simulink model "DC_motor_control_project"  (R2025a)
settings: Solver=VariableStepAuto  StartTime=0.0  StopTime=10.0  RelTol=1e-3
libraries: simulink x1, spsTriangleGeneratorLib x1
settings Model: Creator=HP  LastModifiedBy=HP

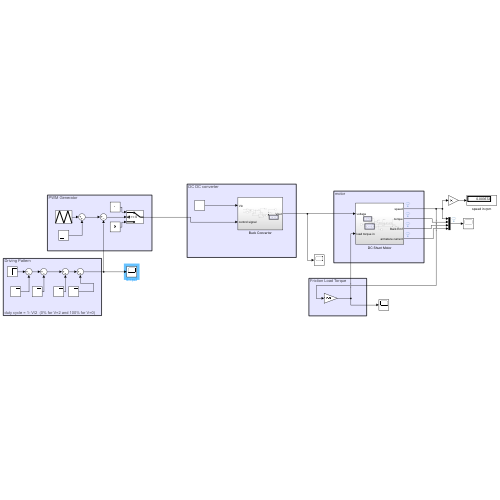
[thumbnail: Simulink's stored preview of the top-level diagram]
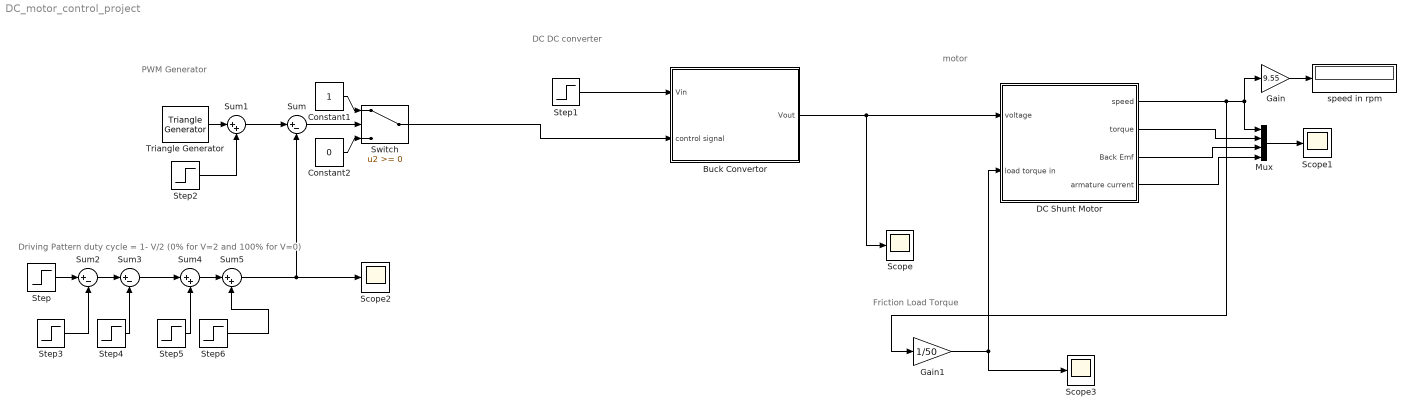
== system DC_motor_control_project ==
  note: motor
  note: Driving Pattern
      |
      |
      |
      |
      |
      |
      |
      |
      |
      |
      | duty cycle = 1- V/2  (0% for V=2 and 100% for V=0)
  note: PWM Generator
  note: DC DC converter
  note: Friction Load Torque
  Buck Convertor : Subsystem
  Constant1 : Constant
  Constant2 : Constant  Value=0
  DC Shunt Motor : Subsystem
  Gain : Gain  Gain=9.55
  Gain1 : Gain  Gain=1/50
  Mux : Mux
  Scope{,1..3} (4 alike) : Scope
      Scope settings: ActiveDisplayYMinimum=-42.370071739541189  ActiveDisplayYMaximum=281.05665253551075  DataLoggingVariableName=ScopeData4
      Scope1 settings: ActiveDisplayYMinimum=-124.79095  ActiveDisplayYMaximum=744.9713
      Scope2 settings: ActiveDisplayYMinimum=-0.24999999999999994  ActiveDisplayYMaximum=2.25  DataLoggingVariableName=ScopeData5
      Scope3 settings: ActiveDisplayYMinimum=-1.8285380504812083  ActiveDisplayYMaximum=16.456842454330879  DataLoggingVariableName=ScopeData6
  Step : Step  Time=0  SampleTime=0
  Step1 : Step  Time=0  After=240  SampleTime=0
  Step2 : Step  Time=0  SampleTime=0
  Step3 : Step  After=0.5  SampleTime=0
  Step4 : Step  Time=2  After=0.5  SampleTime=0
  Step5 : Step  Time=3  After=1.5  SampleTime=0
  Step6 : Step  Time=4  After=0.5  SampleTime=0
  Sum : Sum  Inputs=|+-
  Sum1 : Sum  Inputs=|++
  Sum2 : Sum  Inputs=|+-
  Sum3 : Sum  Inputs=|+-
  Sum4 : Sum  Inputs=|++
  Sum5 : Sum  Inputs=|++
  Switch : Switch  SaturateOnIntegerOverflow=off  InputSameDT=off
  Triangle Generator : spsTriangleGeneratorLib/Triangle Generator  Freq=1e3  Phase=0  Ts=0
  speed in rpm : Display
  wires:
  DC Shunt Motor/4(armature current) -> Mux/4
  DC Shunt Motor/1(speed) -> Gain1/1, Mux/1, Gain/1
  Step1/1 -> Buck Convertor/1(Vin)
  DC Shunt Motor/3(Back Emf) -> Mux/3
  Triangle Generator/1 -> Sum1/1
  Step3/1 -> Sum2/2
  Buck Convertor/1(Vout) -> Scope/1, DC Shunt Motor/1(voltage)
  Step6/1 -> Sum5/2
  Step/1 -> Sum2/1
  Gain/1 -> speed in rpm/1
  Sum3/1 -> Sum4/1
  Sum4/1 -> Sum5/1
  Mux/1 -> Scope1/1
  Constant1/1 -> Switch/1
  Step2/1 -> Sum1/2
  Sum2/1 -> Sum3/1
  Gain1/1 -> DC Shunt Motor/2(load torque in), Scope3/1
  Switch/1 -> Buck Convertor/2(control signal)
  Step5/1 -> Sum4/2
  Constant2/1 -> Switch/3
  Sum5/1 -> Scope2/1, Sum/2
  Sum/1 -> Switch/2
  Step4/1 -> Sum3/2
  Sum1/1 -> Sum/1
  DC Shunt Motor/2(torque) -> Mux/2

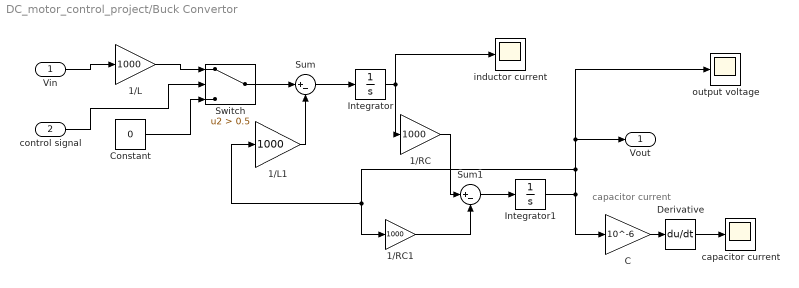
== system DC_motor_control_project/Buck Convertor ==
  note: capacitor current
  Vin : Inport
  control signal : Inport  Port=2
  1/L : Gain  Gain=1000
  1/L1 : Gain  Gain=1000
  1/RC : Gain  Gain=1000
  1/RC1 : Gain  Gain=1000
  C : Gain  Gain=10^-6
  Constant : Constant  Value=0
  Derivative : Derivative
  Integrator : Integrator
  Integrator1 : Integrator
  Sum : Sum  Inputs=|+-
  Sum1 : Sum  Inputs=|+-
  Switch : Switch  Criteria=u2 > Threshold  Threshold=0.5  SaturateOnIntegerOverflow=off  InputSameDT=off
  capacitor current : Scope
      settings: ActiveDisplayYMinimum=-0.14224  ActiveDisplayYMaximum=0.11943  DataLoggingVariableName=ScopeData2
  inductor current : Scope
      settings: ActiveDisplayYMinimum=-52.93589  ActiveDisplayYMaximum=290.861
  output voltage : Scope
      settings: ActiveDisplayYMinimum=-30  ActiveDisplayYMaximum=270  DataLoggingVariableName=ScopeData7
  Vout : Outport
  wires:
  1/L/1 -> Switch/1
  Switch/1 -> Sum/1
  Vin/1 -> 1/L/1
  1/L1/1 -> Sum/2
  Constant/1 -> Switch/3
  Sum/1 -> Integrator/1
  Integrator/1 -> inductor current/1, 1/RC/1
  1/RC/1 -> Sum1/1
  1/RC1/1 -> Sum1/2
  Sum1/1 -> Integrator1/1
  Integrator1/1 -> C/1, 1/L1/1, 1/RC1/1, output voltage/1, Vout/1
  control signal/1 -> Switch/2
  C/1 -> Derivative/1
  Derivative/1 -> capacitor current/1

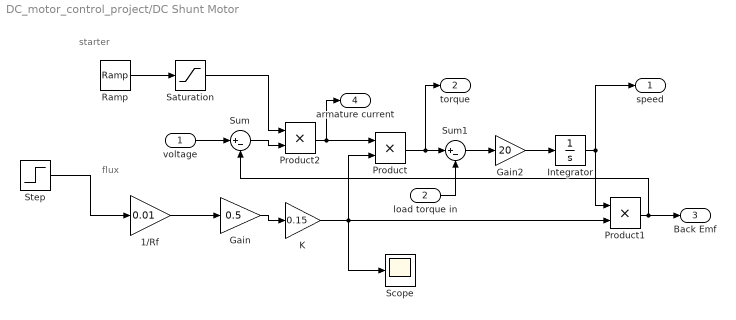
== system DC_motor_control_project/DC Shunt Motor ==
  note: starter
  note: flux
  voltage : Inport
  load torque in : Inport  Port=2
  1/Rf : Gain  Gain=0.01
  Gain : Gain  Gain=0.5
  Gain2 : Gain  Gain=20
  Integrator : Integrator
  K : Gain  Gain=0.15
  Product : Product
  Product1 : Product
  Product2 : Product
  Ramp : simulink/Sources/Ramp  slope=0.5  start=0  InitialOutput=0
  Saturation : Saturate  UpperLimit=5  LowerLimit=0.01
  Scope : Scope
      settings: ActiveDisplayYMinimum=0.065  ActiveDisplayYMaximum=0.265  DataLoggingVariableName=ScopeData3
  Step : Step  Time=0  After=220  SampleTime=0
  Sum : Sum  Inputs=|+-
  Sum1 : Sum  Inputs=|+-
  speed : Outport
  torque : Outport  Port=2
  Back Emf : Outport  Port=3
  armature current : Outport  Port=4
  wires:
  Gain/1 -> K/1
  Sum/1 -> Product2/2
  Product2/1 -> armature current/1, Product/1
  K/1 -> Scope/1, Product/2, Product1/2
  Product/1 -> torque/1, Sum1/1
  load torque in/1 -> Sum1/2
  Sum1/1 -> Gain2/1
  Gain2/1 -> Integrator/1
  Integrator/1 -> speed/1, Product1/1
  Product1/1 -> Back Emf/1, Sum/2
  Ramp/1 -> Saturation/1
  1/Rf/1 -> Gain/1
  voltage/1 -> Sum/1
  Saturation/1 -> Product2/1
  Step/1 -> 1/Rf/1
